simulink model "VREP_controller2018a"  (R2018b)
settings: Solver=FixedStepDiscrete  StartTime=0  StopTime=21  FixedStep=0.005  MaxStep=0.010  RelTol=1e-3  EnableMultiTasking=on
InitFcn:
  | clear all
  | clc
  | 
  | global clientID
  | global vrep
  | global vecJoints nJoints
  | 
  | load_path
  | 
  | 
  | addpath('C:\Program Files\V-REP3\V-REP_PRO_EDU\programming\remoteApiBindings\lib\lib\Windows\64Bit')
  | 
  | 
  | disp('Program started');
  | vrep=remApi('remoteApi'); % using the prototype file (remoteApiProto.m)
  | vrep.simxFinish(-1); % just in case, close all opened connections
  | clientID=vrep.simxStart('127.0.0.1',19997,true,true,5000,5);
  | 
  | vrep.simxStartSimulation(clientID,vrep.simx_opmode_oneshot_wait);
  | vrep.simxSynchronous(clientID,true)
  | 
  | if (clientID<=-1)
  |     disp('stop simulation')
  |     vrep.delete();
  |     set_param(gcs, 'SimulationCommand', 'stop')
  | end
  | 
  | % Root of the joint in Vrep
  | rootJoints     = 'LBR4p_joint';
  | 
  | % Number of joints
  | nJoints        = 7;
  | 
  | % Handles of the joints
  | vecJoints      = zeros(nJoints,1);
  | 
  | for i=1:nJoints
  |                 [res,obj]=vrep.simxGetObjectHandle(clientID,strcat(rootJoints,int2str(i)),vrep.simx_opmode_oneshot_wait);
  |                 if res==vrep.simx_return_ok
  |                     vecJoints(i) = obj;
  |                    [res,pos] = vrep.simxGetJointPosition(clientID,vecJoints(i),vrep.simx_opmode_streaming);
  |                 else
  |                     vecJoints(i) = -1;
  |                     disp(strcat('joint nr ', int2str(i), ' named ', rootJoints, int2str(i) , ' not avalaible!'));
  |                 end
  | end
StopFcn:
  | global clientID
  | 
  | vrep.simxStopSimulation(clientID,vrep.simx_opmode_oneshot_wait);
settings Model: Creator=Massimo  LastModifiedBy=Matteo
settings DataIOCC: LimitDataPoints=on  SaveFormat=Array
settings OptimizationCC: LifeSpan=inf
settings DebuggingCC: UnderspecifiedInitializationDetection=Classic  MergeDetectMultiDrivingBlocksExec=none  StateNameClashWarn=warning  LibraryContextMissingDiagnostic=none  SFUnexpectedBacktrackingDiag=warning  SFNoUnconditionalDefaultTransitionDiag=warning  SFExecutionAtInitializationDiag=none
settings HardwareCC: ProdBitPerPointer=32  ProdBitPerSizeT=32  ProdBitPerPtrDiffT=32  ProdLargestAtomicFloat=None  ProdIntDivRoundTo=Undefined  ProdEndianess=Unspecified  ProdWordSize=32  ProdHWDeviceType=32-bit Generic
settings ModelReferenceCC: PropagateSignalLabelsOutOfModel=off
settings SFSimCC: SimUseLocalCustomCode=off
settings RTWCC: RTWUseLocalCustomCode=off
settings CodeAppCC: StateflowObjectComments=on
settings GRTTargetCC: TargetLangStandard=C89/C90 (ANSI)  GeneratePreprocessorConditionals=Disable all
settings ConfigComp: CovMetricSettings=dw  CovHtmlReporting=on  CovSaveCumulativeToWorkspaceVar=on  CovSaveSingleToWorkspaceVar=on  CovExternalEMLEnable=off

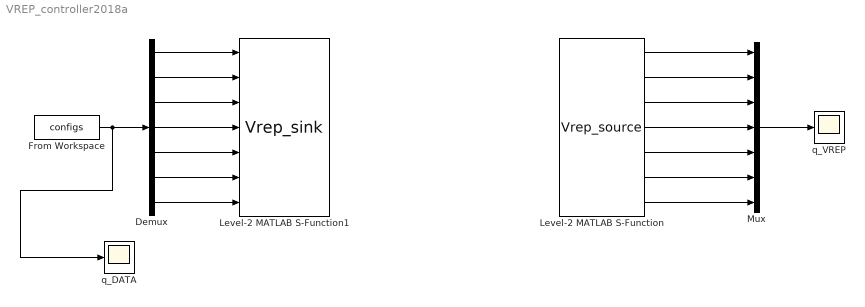
== system VREP_controller2018a ==
  Demux : Demux  Outputs=7
  From Workspace : FromWorkspace  VariableName=configs  OutDataTypeStr=double  SampleTime=0
  Level-2 MATLAB S-Function : M-S-Function  FunctionName=Vrep_source
  Level-2 MATLAB S-Function1 : M-S-Function  FunctionName=Vrep_sink
  Mux : Mux  Inputs=7
  q_DATA : Scope
  q_VREP : Scope
  wires:
  From Workspace/1 -> q_DATA/1, Demux/1
  Demux/4 -> Level-2 MATLAB S-Function1/4
  Demux/5 -> Level-2 MATLAB S-Function1/5
  Demux/3 -> Level-2 MATLAB S-Function1/3
  Demux/2 -> Level-2 MATLAB S-Function1/2
  Demux/1 -> Level-2 MATLAB S-Function1/1
  Demux/6 -> Level-2 MATLAB S-Function1/6
  Demux/7 -> Level-2 MATLAB S-Function1/7
  Level-2 MATLAB S-Function/4 -> Mux/4
  Level-2 MATLAB S-Function/3 -> Mux/3
  Level-2 MATLAB S-Function/2 -> Mux/2
  Level-2 MATLAB S-Function/1 -> Mux/1
  Level-2 MATLAB S-Function/5 -> Mux/5
  Level-2 MATLAB S-Function/6 -> Mux/6
  Level-2 MATLAB S-Function/7 -> Mux/7
  Mux/1 -> q_VREP/1
